simulink subsystem "DC_Machine_Model"  (R2023a)
settings: Solver=VariableStepAuto  StartTime=0.0  StopTime=10.0  RelTol=1e-3
undefined symbols (not defined in the file): J, Km, La, Lf, Ra, Rf
libraries: spsCurrentMeasurementLib x2, spsSeriesRLCBranchLib x2, spsControlledVoltageSourceLib x1
settings Model: Creator=gaming3  LastModifiedBy=gaming3

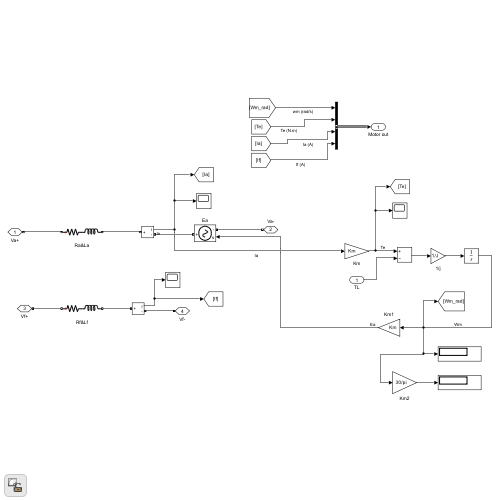
[thumbnail: Simulink's stored preview of the top-level diagram]
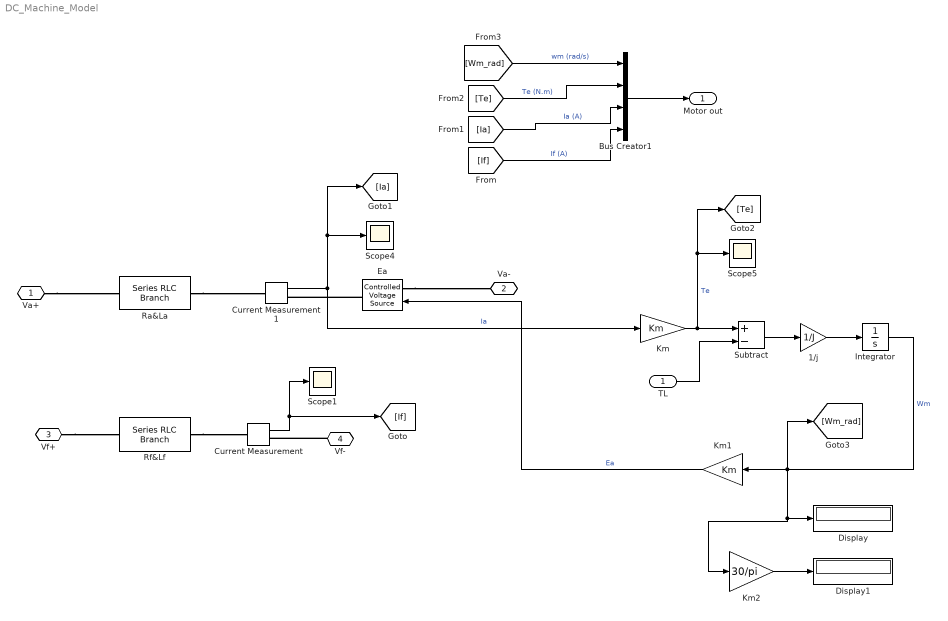
== system DC_Machine_Model ==
  TL : Inport
  1/j : Gain  Gain=1/J
  Bus Creator1 : BusCreator  Inputs=4
  Current Measurement : spsCurrentMeasurementLib/Current Measurement  PhasorSimulation=off  OutputType=Complex  PSBequivalent=0
  Current Measurement1 : spsCurrentMeasurementLib/Current Measurement  PhasorSimulation=off  OutputType=Complex  PSBequivalent=0
  Display : Display
  Display1 : Display
  Ea : spsControlledVoltageSourceLib/Controlled Voltage Source  Initialize=on  Source_Type=AC  Amplitude=0  Phase=0  Frequency=0  Measurements=None
  Integrator : Integrator
  Km : Gain  Gain=Km
  Km1 : Gain  Gain=Km
  Km2 : Gain  Gain=30/pi
  Ra&La : spsSeriesRLCBranchLib/Series RLC Branch  LConnTagsString=__new0  RConnTagsString=__new0  BranchType=RL  Resistance=Ra  Inductance=La  SetiL0=off  InitialCurrent=0  Capacitance=1e-6  Setx0=off  InitialVoltage=0  Measurements=None
  Rf&Lf : spsSeriesRLCBranchLib/Series RLC Branch  LConnTagsString=__new0  RConnTagsString=__new0  BranchType=RL  Resistance=Rf  Inductance=Lf  SetiL0=off  InitialCurrent=0  Capacitance=1e-6  Setx0=off  InitialVoltage=0  Measurements=None
  Scope1 : Scope
  Scope4 : Scope
  Scope5 : Scope
  Subtract : Sum  Inputs=+-
  Va+ : PMIOPort  Side=Left
  Va- : PMIOPort  Port=2  Side=Right
  Vf+ : PMIOPort  Port=3  Side=Left
  Vf- : PMIOPort  Port=4  Side=Right
  Motor out : Outport
  wires:
  Km/1 -> Subtract/1, Scope5/1, [Te]  "Te"
  1/j/1 -> Integrator/1
  Current Measurement/1 -> [If], Scope1/1
  Integrator/1 -> Km1/1, Display/1, Km2/1, [Wm_rad]  "Wm"
  Km2/1 -> Display1/1
  Current Measurement1/1 -> Km/1, Scope4/1, [Ia]  "Ia"
  Subtract/1 -> 1/j/1
  TL/1 -> Subtract/2
  Km1/1 -> Ea/1  "Ea"
  Bus Creator1/1 -> Motor out/1
  [Wm_rad] -> Bus Creator1/1  "wm (rad/s)"
  [Te] -> Bus Creator1/2  "Te (N.m)"
  [Ia] -> Bus Creator1/3  "Ia (A)"
  [If] -> Bus Creator1/4  "If (A)"
  connections:
  Va+/RConn1 -- Ra&La/LConn1
  Rf&Lf/RConn1 -- Current Measurement/LConn1
  Ea/RConn1 -- Current Measurement1/RConn1
  Ra&La/RConn1 -- Current Measurement1/LConn1
  Vf-/RConn1 -- Current Measurement/RConn1
  Ea/LConn1 -- Va-/RConn1
  Vf+/RConn1 -- Rf&Lf/LConn1
